simulink model "MATLAB_Task"  (R2024a)
settings: Solver=VariableStepAuto  StartTime=0.0  StopTime=15  RelTol=1e-3
libraries: spsRMSLib x9, spsThreePhaseVIMeasurementLib x6, spsThreePhaseTransformerTwoWindingsLib x4, spsThreePhaseBreakerLib x2, spsThreePhaseParallelRLCLoadLib x2, spsThreePhaseSourceLib x2, spsPowerLib x1, spsThreePhasePISectionLineLib x1, sps_lib x1
settings Model: Creator=samee  LastModifiedBy=samee

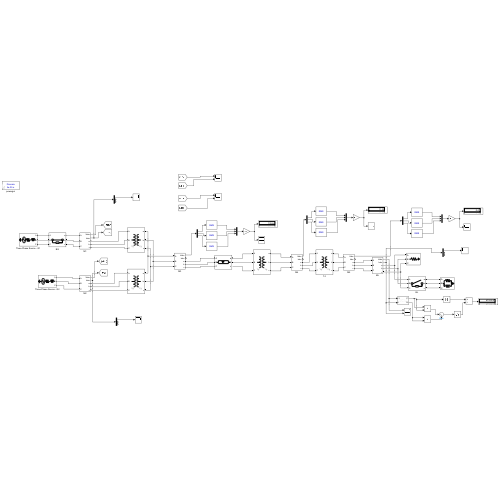
[thumbnail: Simulink's stored preview of the top-level diagram]
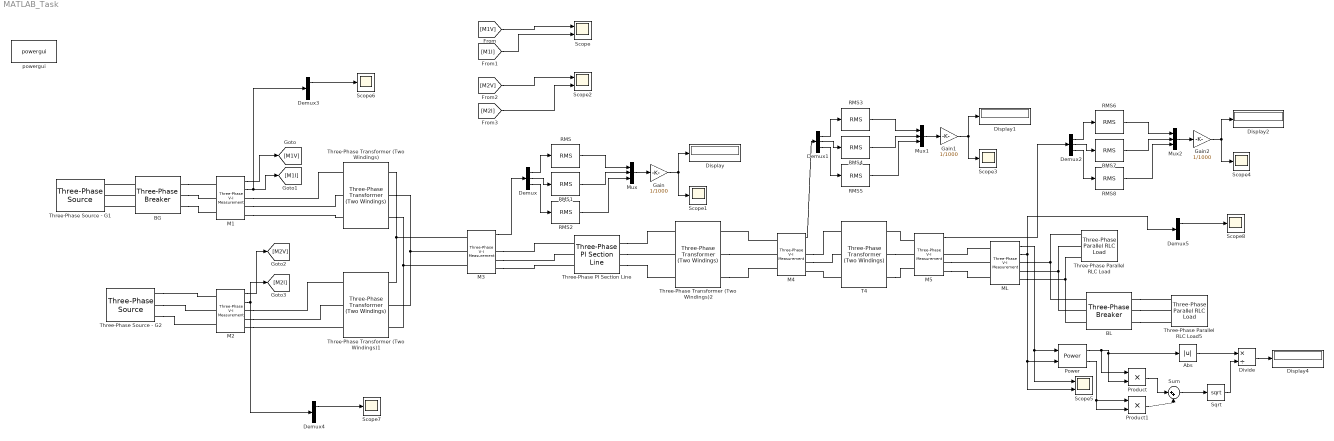
== system MATLAB_Task ==
  Abs : Abs  SaturateOnIntegerOverflow=off
  BG : spsThreePhaseBreakerLib/Three-Phase Breaker  InitialState=closed  SwitchA=on  SwitchB=on  SwitchC=on  SwitchTimes=[10]  External=off  BreakerResistance=0.001  SnubberResistance=1e6  SnubberCapacitance=inf  Measurements=None
  BL : spsThreePhaseBreakerLib/Three-Phase Breaker  InitialState=open  SwitchA=on  SwitchB=on  SwitchC=on  SwitchTimes=[5]  External=off  BreakerResistance=0.001  SnubberResistance=1e6  SnubberCapacitance=inf  Measurements=None
  Demux{,1..5} (6 alike) : Demux  Outputs=3
  Display{,1..2,4} (4 alike) : Display
      settings: Format=bank
  Divide : Product  Inputs=*/
  Gain : Gain  Gain=1/1000
  Gain1 : Gain  Gain=1/1000
  Gain2 : Gain  Gain=1/1000
  M{1..5} (5 alike) : spsThreePhaseVIMeasurementLib/Three-Phase V-I Measurement  VoltageMeasurement=phase-to-phase  SetLabelV=off  LabelV=Vabc  Vpu=off  VpuLL=off  CurrentMeasurement=yes  SetLabelI=off  LabelI=Iabc  Ipu=off  Pbase=100e6  Vbase=500e3  OutputType=Complex  PhasorSimulation=off  PSBequivalent=0
  ML : spsThreePhaseVIMeasurementLib/Three-Phase V-I Measurement  VoltageMeasurement=phase-to-ground  SetLabelV=off  LabelV=Vabc  Vpu=off  VpuLL=off  CurrentMeasurement=yes  SetLabelI=off  LabelI=Iabc  Ipu=off  Pbase=100e6  Vbase=500e3  OutputType=Complex  PhasorSimulation=off  PSBequivalent=0
  Mux : Mux  Inputs=3
  Mux1 : Mux  Inputs=3
  Mux2 : Mux  Inputs=3
  Power : spsPowerLib/Power  Freq=60  Vinit=[1, 0]  Iinit=[1, 0]  Ts=0
  Product : Product
  Product1 : Product
  RMS{,1..8} (9 alike) : spsRMSLib/RMS  TrueRMS=on  Freq=50  RMSInit=120  Ts=0
  Scope : Scope  NumInputPorts=2
  Scope{1,3..4,6..8} (6 alike) : Scope
  Scope2 : Scope  NumInputPorts=2
  Scope5 : Scope  NumInputPorts=2
  Sqrt : Sqrt
  Sum : Sum  Inputs=|++
  T4 : spsThreePhaseTransformerTwoWindingsLib/Three-Phase Transformer (Two Windings)  Winding1Connection=Yg  Winding2Connection=Yg  CoreType=Three single-phase transformers  SetSaturation=off  Hysteresis=off  DataFile='hysteresis'  SetInitialFlux=off  Measurements=None  UNITS=pu  NominalPower=[ 5e6 , 50 ]  Winding1=[ 11e3 , 0.005 , 0.02 ]  Winding2=[ 400 , 0.005 , 0.02 ]  Rm=500  Lm=500  L0=0.5  Saturation=[ 0,0 ; 0.0024,1.2 ; 1.0,1.52 ]  InitialFluxes=[ 0.8 , -0.8 , 0.7 ]  BreakLoop=off  DiscreteSolver=Trapezoidal iterative  DataType=off  TransfoNumber=1
  Three-Phase PI Section Line : spsThreePhasePISectionLineLib/Three-Phase PI Section Line  LConnTagsString=a|b|c  RConnTagsString=A|B|C  Length=50  Frequency=50  Resistances=[ 0.01273 0.3864]  Inductances="[ 0.9337e-3  4.1264e-3]"  Capacitances=[12.74e-9 7.751e-9]
  Three-Phase Parallel RLC Load : spsThreePhaseParallelRLCLoadLib/Three-Phase Parallel RLC Load  LConnTagsString=A|B|C  Configuration=Y (grounded)  NominalVoltage=400  Vabc=[1e3 1e3 1e3]  Vabcp=[1e3 1e3 1e3]  NominalFrequency=50  UnbalancedPower=off  ActivePower=575e3  InductivePower=0  CapacitivePower=0  Pabc=[10e3 9e3 11e3]  QLabc=[100 90 110]  QCabc=[100 90 110]  Pabcp=[10e3 9e3 11e3]  QLabcp=[100 90 110]  QCabcp=[100 90 110]  Measurements=None  LoadType=constant Z
  Three-Phase Parallel RLC Load5 : spsThreePhaseParallelRLCLoadLib/Three-Phase Parallel RLC Load  LConnTagsString=A|B|C  Configuration=Y (grounded)  NominalVoltage=400  Vabc=[1e3 1e3 1e3]  Vabcp=[1e3 1e3 1e3]  NominalFrequency=50  UnbalancedPower=off  ActivePower=285e3  InductivePower=213750  CapacitivePower=0  Pabc=[10e3 9e3 11e3]  QLabc=[100 90 110]  QCabc=[100 90 110]  Pabcp=[10e3 9e3 11e3]  QLabcp=[100 90 110]  QCabcp=[100 90 110]  Measurements=None  LoadType=constant Z
  Three-Phase Transformer (Two Windings) : spsThreePhaseTransformerTwoWindingsLib/Three-Phase Transformer (Two Windings)  Winding1Connection=Yg  Winding2Connection=Yg  CoreType=Three single-phase transformers  SetSaturation=off  Hysteresis=off  DataFile='hysteresis'  SetInitialFlux=off  Measurements=None  UNITS=pu  NominalPower=[ 5e6 , 50 ]  Winding1=[ 6.5e3 , 0.005 , 0.02 ]  Winding2=[ 132e3 , 0.005 , 0.02 ]  Rm=500  Lm=500  L0=0.5  Saturation=[ 0,0 ; 0.0024,1.2 ; 1.0,1.52 ]  InitialFluxes=[ 0.8 , -0.8 , 0.7 ]  BreakLoop=off  DiscreteSolver=Trapezoidal iterative  DataType=off  TransfoNumber=1
  Three-Phase Transformer (Two Windings)1 : spsThreePhaseTransformerTwoWindingsLib/Three-Phase Transformer (Two Windings)  Winding1Connection=Yg  Winding2Connection=Yg  CoreType=Three single-phase transformers  SetSaturation=off  Hysteresis=off  DataFile='hysteresis'  SetInitialFlux=off  Measurements=None  UNITS=pu  NominalPower=[ 10e6 , 50 ]  Winding1=[ 11e3 , 0.005 , 0.02 ]  Winding2=[ 132e3 , 0.005 , 0.02 ]  Rm=500  Lm=500  L0=0.5  Saturation=[ 0,0 ; 0.0024,1.2 ; 1.0,1.52 ]  InitialFluxes=[ 0.8 , -0.8 , 0.7 ]  BreakLoop=off  DiscreteSolver=Trapezoidal iterative  DataType=off  TransfoNumber=1
  Three-Phase Transformer (Two Windings)2 : spsThreePhaseTransformerTwoWindingsLib/Three-Phase Transformer (Two Windings)  Winding1Connection=Yg  Winding2Connection=Yg  CoreType=Three single-phase transformers  SetSaturation=off  Hysteresis=off  DataFile='hysteresis'  SetInitialFlux=off  Measurements=None  UNITS=pu  NominalPower=[ 15e6 , 50 ]  Winding1=[ 132e3 , 0.005 , 0.02 ]  Winding2=[ 11e3 , 0.005 , 0.02 ]  Rm=500  Lm=500  L0=0.5  Saturation=[ 0,0 ; 0.0024,1.2 ; 1.0,1.52 ]  InitialFluxes=[ 0.8 , -0.8 , 0.7 ]  BreakLoop=off  DiscreteSolver=Trapezoidal iterative  DataType=off  TransfoNumber=1
  Three-Phase Source - G1 : spsThreePhaseSourceLib/Three-Phase Source  InternalConnection=Yg  VoltagePhases=off  Voltage=6500  PhaseAngle=0  Voltage_phases=[25e3 25e3 25e3]/sqrt(3)  PhaseAngles_phases=[0 -120 +120]  Frequency=50  NonIdealSource=on  SpecifyImpedance=off  Resistance=0.2  Inductance=0.002  ShortCircuitLevel=100e6  BaseVoltage=25e3  XRratio=7  BusType=swing  Pref=10e3  Qref=0  Prefabc=[10e3, 10e3, 10e3]  Qrefabc=[0, 0, 0]  Qmin=-inf  Qmax=inf
  Three-Phase Source - G2 : spsThreePhaseSourceLib/Three-Phase Source  InternalConnection=Yg  VoltagePhases=off  Voltage=11000  PhaseAngle=0  Voltage_phases=[25e3 25e3 25e3]/sqrt(3)  PhaseAngles_phases=[0 -120 +120]  Frequency=50  NonIdealSource=on  SpecifyImpedance=off  Resistance=0.2  Inductance=0.002  ShortCircuitLevel=100e6  BaseVoltage=25e3  XRratio=7  BusType=swing  Pref=10e3  Qref=0  Prefabc=[10e3, 10e3, 10e3]  Qrefabc=[0, 0, 0]  Qmin=-inf  Qmax=inf
  powergui : sps_lib/powergui  Priority=1  SimulationMode=Discrete  SampleTime=5e-5  frequency=60  Iterations=50  frequencyindice=50  Pbase=100e6  ErrMax=1e-4  UnitsV=kV  UnitsW=MW  buscounter=0  FunctionMessages=off  echomessages=off  EnableUseOfTLC=off  CurrentSourceSwitches=off  DisableSnubberDevices=off  DisableRonSwitches=off  DisableVfSwitches=off  DisplayEquations=off  AutomaticDiscreteSolvers=off  SolverType=Tustin/Backward Euler (TBE)  Interpol=off  ExternalGateDelay=off  methode=off  Ts=100  x0status=blocks  SPID=on  SwTol=0  HookPort=off  NonlinearTolerance=1e-4  nMaxIteration=100  ContinueOnMaxIteration=off  RestoreLinks=warning  ResistiveCurrentMeasurement=off  Frange=[0:2:500]  Ylog=off  Xlog=on  ShowGrid=off  save=off  variable=ZData  structure=0  ZoomFFT=off  StartTime=0.0  cycles=1  DisplayStyle=1  fundamental=60  FreqAxis=off  MaxFrequency=1000  frequencyindicesteady=1  RmsSteady=1  display=off
  wires:
  M1/1 -> [M1V]
  M1/2 -> Demux3/1, [M1I]
  [M1V] -> Scope/1
  [M1I] -> Scope/2
  M2/1 -> [M2V]
  M2/2 -> Demux4/1, [M2I]
  [M2V] -> Scope2/1
  [M2I] -> Scope2/2
  M3/1 -> Demux/1
  Demux/1 -> RMS/1
  Demux/3 -> RMS2/1
  Demux/2 -> RMS1/1
  RMS/1 -> Mux/1
  RMS1/1 -> Mux/2
  RMS2/1 -> Mux/3
  Mux/1 -> Gain/1
  Gain/1 -> Scope1/1, Display/1
  Mux1/1 -> Gain1/1
  Demux1/3 -> RMS5/1
  RMS3/1 -> Mux1/1
  Demux1/2 -> RMS4/1
  Demux1/1 -> RMS3/1
  RMS4/1 -> Mux1/2
  RMS5/1 -> Mux1/3
  Gain1/1 -> Scope3/1, Display1/1
  M4/1 -> Demux1/1
  Gain2/1 -> Scope4/1, Display2/1
  RMS6/1 -> Mux2/1
  Mux2/1 -> Gain2/1
  RMS8/1 -> Mux2/3
  Demux2/3 -> RMS8/1
  Demux2/1 -> RMS6/1
  RMS7/1 -> Mux2/2
  Demux2/2 -> RMS7/1
  M5/1 -> Demux2/1
  ML/1 -> Power/1, Scope5/1
  ML/2 -> Demux5/1, Scope5/2, Power/2
  Power/1 -> Product/1, Product/2, Abs/1
  Power/2 -> Product1/2, Product1/1
  Product/1 -> Sum/1
  Product1/1 -> Sum/2
  Sum/1 -> Sqrt/1
  Abs/1 -> Divide/1
  Sqrt/1 -> Divide/2
  Divide/1 -> Display4/1
  Demux3/1 -> Scope6/1
  Demux4/1 -> Scope7/1
  Demux5/1 -> Scope8/1
  connections:
  Three-Phase Source - G2/RConn1 -- M2/LConn1
  Three-Phase Source - G2/RConn2 -- M2/LConn2
  Three-Phase Source - G2/RConn3 -- M2/LConn3
  M1/RConn1 -- Three-Phase Transformer (Two Windings)/LConn1
  M1/RConn2 -- Three-Phase Transformer (Two Windings)/LConn2
  M1/RConn3 -- Three-Phase Transformer (Two Windings)/LConn3
  M2/RConn1 -- Three-Phase Transformer (Two Windings)1/LConn1
  M2/RConn2 -- Three-Phase Transformer (Two Windings)1/LConn2
  M2/RConn3 -- Three-Phase Transformer (Two Windings)1/LConn3
  Three-Phase PI Section Line/RConn1 -- Three-Phase Transformer (Two Windings)2/LConn1
  Three-Phase PI Section Line/RConn2 -- Three-Phase Transformer (Two Windings)2/LConn2
  Three-Phase PI Section Line/RConn3 -- Three-Phase Transformer (Two Windings)2/LConn3
  Three-Phase Transformer (Two Windings)/RConn1 -- Three-Phase Transformer (Two Windings)1/RConn1 -- M3/LConn1
  Three-Phase Transformer (Two Windings)/RConn2 -- M3/LConn2 -- Three-Phase Transformer (Two Windings)1/RConn2
  Three-Phase Transformer (Two Windings)/RConn3 -- M3/LConn3 -- Three-Phase Transformer (Two Windings)1/RConn3
  M3/RConn1 -- Three-Phase PI Section Line/LConn1
  M3/RConn2 -- Three-Phase PI Section Line/LConn2
  M3/RConn3 -- Three-Phase PI Section Line/LConn3
  M4/LConn1 -- Three-Phase Transformer (Two Windings)2/RConn1
  Three-Phase Transformer (Two Windings)2/RConn2 -- M4/LConn2
  Three-Phase Transformer (Two Windings)2/RConn3 -- M4/LConn3
  M5/LConn1 -- T4/RConn1
  T4/RConn2 -- M5/LConn2
  T4/RConn3 -- M5/LConn3
  BG/LConn1 -- Three-Phase Source - G1/RConn1
  BG/LConn2 -- Three-Phase Source - G1/RConn2
  BG/LConn3 -- Three-Phase Source - G1/RConn3
  BG/RConn1 -- M1/LConn1
  BG/RConn2 -- M1/LConn2
  BG/RConn3 -- M1/LConn3
  ML/LConn1 -- M5/RConn1
  M5/RConn2 -- ML/LConn2
  M5/RConn3 -- ML/LConn3
  M4/RConn1 -- T4/LConn1
  M4/RConn2 -- T4/LConn2
  T4/LConn3 -- M4/RConn3
  ML/RConn1 -- BL/LConn1 -- Three-Phase Parallel RLC Load/LConn1
  ML/RConn2 -- BL/LConn2 -- Three-Phase Parallel RLC Load/LConn2
  ML/RConn3 -- BL/LConn3 -- Three-Phase Parallel RLC Load/LConn3
  BL/RConn1 -- Three-Phase Parallel RLC Load5/LConn1
  BL/RConn2 -- Three-Phase Parallel RLC Load5/LConn2
  BL/RConn3 -- Three-Phase Parallel RLC Load5/LConn3
